simulink model "ON_ALARM"  (R2022b)
settings: Solver=FixedStepDiscrete  StartTime=0.0  StopTime=10.0  FixedStep=0.1  RelTol=1e-3  EnableMultiTasking=on
settings Model: DVExtractedSubsystem=ON.ALARM  Creator=alewi  LastModifiedBy=alewi
settings SolverCC: AlgebraicLoopSolver=TrustRegion  AutoInsertRateTranBlk=on
settings DataIOCC: LimitDataPoints=on
settings OptimizationCC: LifeSpan=inf
settings DebuggingCC: UnconnectedInputMsg=warning  UnconnectedOutputMsg=warning  UnconnectedLineMsg=warning  FrameProcessingCompatibilityMsg=none  AllowSymbolicDim=off  SFUnexpectedBacktrackingDiag=warning  SFNoUnconditionalDefaultTransitionDiag=warning  SFExecutionAtInitializationDiag=none  ArithmeticOperatorsInVariantConditions=warning
settings ModelReferenceCC: EnableRefExpFcnMdlSchedulingChecks=on
settings SFSimCC: SimUseLocalCustomCode=off  CustomCodeUndefinedFunction=UseInterfaceOnly
settings RTWCC: TLCOptions=-aAlwaysIncludeCustomSrc=1  RTWUseLocalCustomCode=off  DLArmComputeVersion=19.05
settings CodeAppCC: StateflowObjectComments=on
settings GRTTargetCC: TargetLangStandard=C89/C90 (ANSI)
settings ConfigComp: CovMetricSettings=dw  CovSaveCumulativeToWorkspaceVar=on  CovSaveSingleToWorkspaceVar=on  CovExternalEMLEnable=off  CovSFcnEnable=off  DVTestSuiteOptimization=Auto  DVDetectOutOfBounds=on  DVModelReferenceHarness=on  DVHarnessSource=Signal Editor

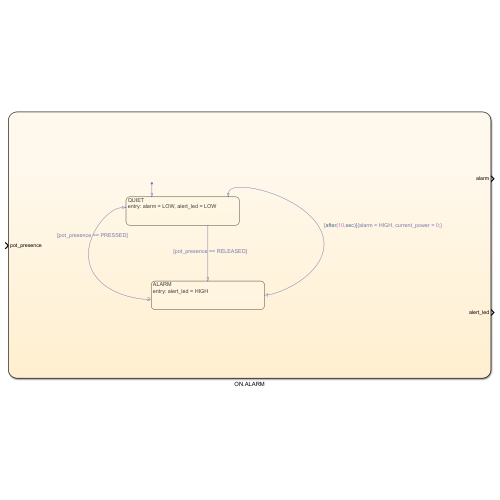
[thumbnail: Simulink's stored preview of the top-level diagram]
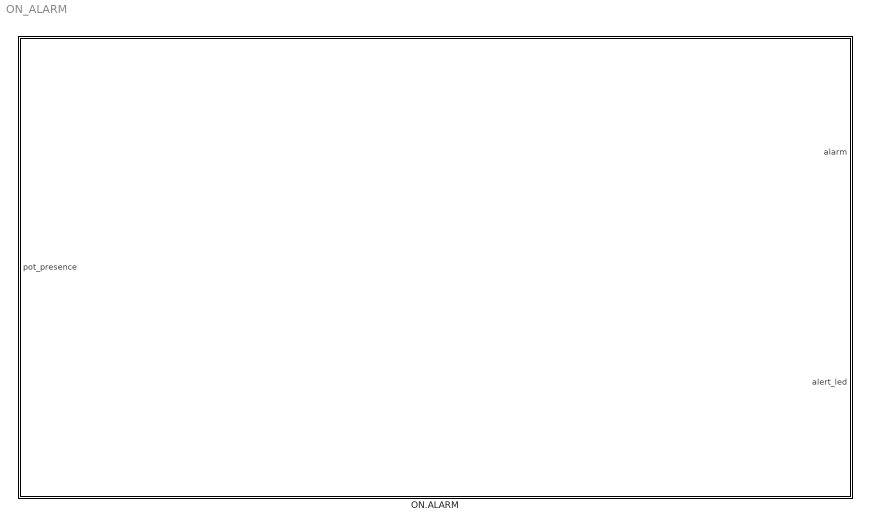
== system ON_ALARM ==
  ON.ALARM : Stateflow chart  Priority=0  TreatAsAtomicUnit=on

== stateflow chart ON_ALARM/ON.ALARM ==
  state QUIET
    entry: alarm = LOW, alert_led = LOW
  state ALARM
    entry: alert_led = HIGH
  (default) -> QUIET
  ALARM -> QUIET [order 1] : [after(10,sec)]{alarm = HIGH, current_power = 0;}
  ALARM -> QUIET [order 2] : [pot_presence == PRESSED]
  QUIET -> ALARM : [pot_presence == RELEASED]
  data: HIGH constant boolean =1; LOW constant boolean =0; PRESSED constant boolean =0; RELEASED constant boolean =1; pot_presence input boolean size=1; alarm output boolean size=1; current_power data_store_memory size=1; alert_led output boolean size=1
